simulink model "untitled"  (R2019a)
settings: Solver=VariableStepAuto  StartTime=0  StopTime=30  FixedStep=0.001  RelTol=1e-3
settings Model: Creator=Me  LastModifiedBy=Me

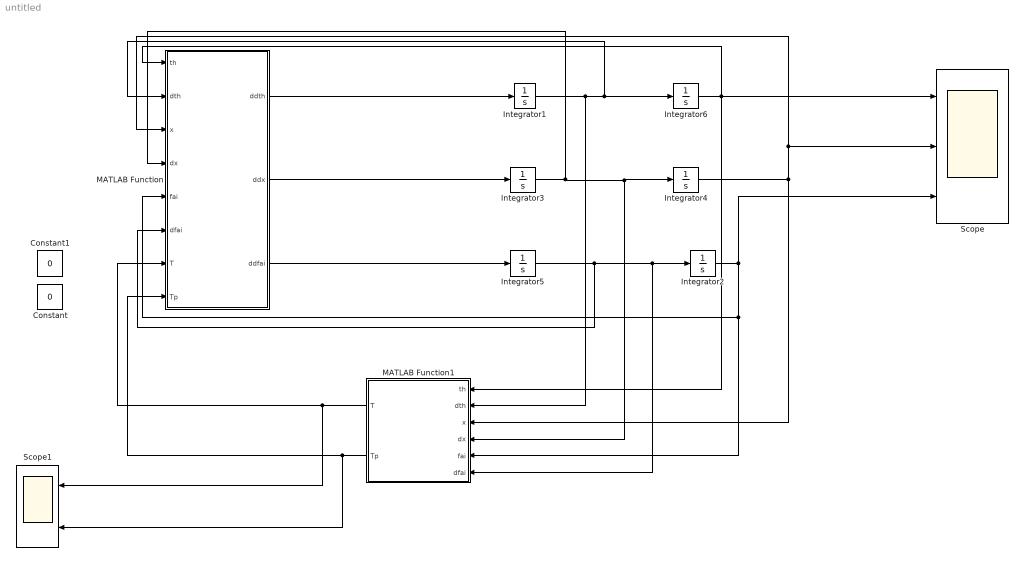
== system untitled ==
  Constant : Constant  Value=0
  Constant1 : Constant  Value=0
  Integrator{1,3..5} (4 alike) : Integrator
  Integrator2 : Integrator  InitialCondition=0.5
  Integrator6 : Integrator  InitialCondition=0.0
  MATLAB Function : MATLAB Function  TreatAsAtomicUnit=on
  MATLAB Function1 : MATLAB Function  TreatAsAtomicUnit=on
  Scope : Scope  NumInputPorts=3
  Scope1 : Scope  NumInputPorts=2
  wires:
  MATLAB Function/1(ddth) -> Integrator1/1
  MATLAB Function/2(ddx) -> Integrator3/1
  MATLAB Function/3(ddfai) -> Integrator5/1
  Integrator1/1 -> Integrator6/1, MATLAB Function/2(dth), MATLAB Function1/2(dth)
  Integrator3/1 -> MATLAB Function/4(dx), MATLAB Function1/4(dx), Integrator4/1
  Integrator5/1 -> MATLAB Function/6(dfai), MATLAB Function1/6(dfai), Integrator2/1
  Integrator6/1 -> MATLAB Function1/1(th), Scope/1, MATLAB Function/1(th)
  Integrator4/1 -> Scope/2, MATLAB Function/3(x), MATLAB Function1/3(x)
  Integrator2/1 -> MATLAB Function1/5(fai), MATLAB Function/5(fai), Scope/3
  MATLAB Function1/1(T) -> Scope1/1, MATLAB Function/7(T)
  MATLAB Function1/2(Tp) -> Scope1/2, MATLAB Function/8(Tp)

== matlab function untitled/MATLAB Function1 ==
  data: th input; T output; dth input; x input; dx input; fai input; dfai input; Tp output
function [T,Tp] = control_LQR(th,dth,x,dx,fai,dfai)

K=[-512.585410082294,-161.955429419996,-1.78875088891739,-4.14450385580597,80.9920408281173,18.7038034389622;-603.700719342304,-190.743677932792,-5.83111064172711,-10.2534853636546,179.718060238728,40.7009819117587];
U=-(K*[th,dth,x,dx,fai,dfai]')';

T=min(max(U(1),-100),100);
Tp=min(max(U(2),-40),40);

== matlab function untitled/MATLAB Function ==
  data: th input; dth input; x input; dx input; fai input; dfai input; T input; Tp input; ddth output; ddx output; ddfai output
function [ddth,ddx,ddfai]=sfuntmpl(th,dth,x,dx,fai,dfai,T, Tp)
R=0.25/2;
L =0.5;  %摆杆重心到驱动轮轴距离
LM =0.5; %摆杆重心到机体转轴距离
l =0.2;  %机体重心到机体转轴距离
mw =1;   %转子质量
mp =2;   %摆杆质量
M=20;    %机体质量
Iw =0.5*mw*(R^2+(R-0.03)^2);%转子惯量
Ip =1/4*mp*0.08^2+1/12*mp*L^2;%摆杆惯量
IM =1/4*M*0.3^2+1/12*M*0.7^2;%机体惯量
g =9.8;


ddfai =(Tp + M*g*l*sin(fai) - L*M*dth^2*l*sin(fai + th) - LM*M*dth^2*l*sin(fai + th))/(M*l^2 + IM);
ddth =(Tp - T + L*M*g*sin(th) + LM*M*g*sin(th) + L*g*mp*sin(th) - L*M*dfai^2*l*sin(fai + th) - LM*M*dfai^2*l*sin(fai + th))/(Ip + L^2*M + LM^2*M + L^2*mp + 2*L*LM*M);
ddx =(T + R*(M*(- l*sin(fai)*dfai^2 + sin(th)*(L + LM)*dth^2) + L*dth^2*mp*sin(th)))/(((R*(M + mp))/(R*mw + Iw/R) + 1)*(R*mw + Iw/R));
